simulink model "electroMagneticModel_SS"  (R2017b)
settings: Solver=VariableStepAuto  StartTime=0.0  StopTime=5  RelTol=1e-3
undefined symbols (not defined in the file): Ax, Bx, Cx, Dx, u_0, x_0
settings Model: Creator=lasse  LastModifiedBy=lasse

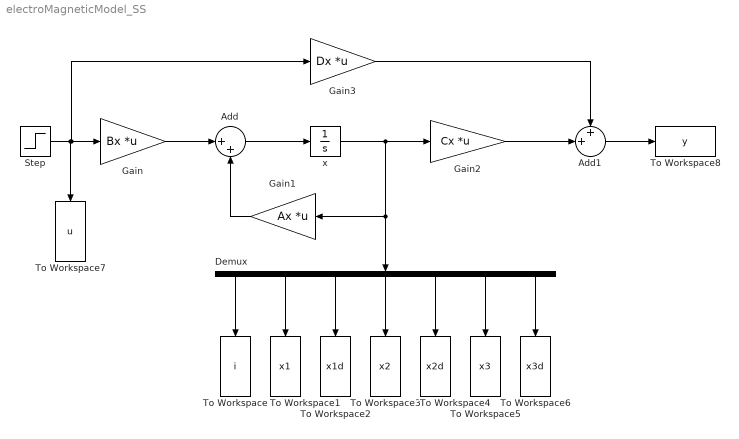
== system electroMagneticModel_SS ==
  Add : Sum  Inputs=|++
  Add1 : Sum  Inputs=++|
  Demux : Demux  Outputs=7
  Gain : Gain  Gain=Bx  Multiplication=Matrix(K*u) (u vector)
  Gain1 : Gain  Gain=Ax  Multiplication=Matrix(K*u) (u vector)
  Gain2 : Gain  Gain=Cx  Multiplication=Matrix(K*u) (u vector)
  Gain3 : Gain  Gain=Dx  Multiplication=Matrix(K*u) (u vector)
  Step : Step  After=u_0  SampleTime=0
  To Workspace : ToWorkspace  VariableName=i  SaveFormat=Structure With Time  SampleTime=-1
  To Workspace1 : ToWorkspace  VariableName=x1  SaveFormat=Structure With Time  SampleTime=-1
  To Workspace2 : ToWorkspace  VariableName=x1d  SaveFormat=Structure With Time  SampleTime=-1
  To Workspace3 : ToWorkspace  VariableName=x2  SaveFormat=Structure With Time  SampleTime=-1
  To Workspace4 : ToWorkspace  VariableName=x2d  SaveFormat=Structure With Time  SampleTime=-1
  To Workspace5 : ToWorkspace  VariableName=x3  SaveFormat=Structure With Time  SampleTime=-1
  To Workspace6 : ToWorkspace  VariableName=x3d  SaveFormat=Structure With Time  SampleTime=-1
  To Workspace7 : ToWorkspace  VariableName=u  SaveFormat=Structure With Time  SampleTime=-1
  To Workspace8 : ToWorkspace  VariableName=y  SaveFormat=Structure With Time  SampleTime=-1
  x : Integrator  InitialCondition=x_0
  wires:
  Step/1 -> Gain3/1, Gain/1, To Workspace7/1
  Gain/1 -> Add/1
  Gain1/1 -> Add/2
  Add/1 -> x/1
  Gain2/1 -> Add1/2
  Gain3/1 -> Add1/1
  x/1 -> Gain1/1, Demux/1, Gain2/1
  Demux/1 -> To Workspace/1
  Demux/3 -> To Workspace2/1
  Demux/2 -> To Workspace1/1
  Demux/4 -> To Workspace3/1
  Demux/5 -> To Workspace4/1
  Demux/6 -> To Workspace5/1
  Demux/7 -> To Workspace6/1
  Add1/1 -> To Workspace8/1
